simulink model "questao1"  (Simulink 3.00)
settings: Solver=ode45  StartTime=0.0  StopTime=4  RelTol=1e-3
settings Model: LastModifiedBy=Administrador

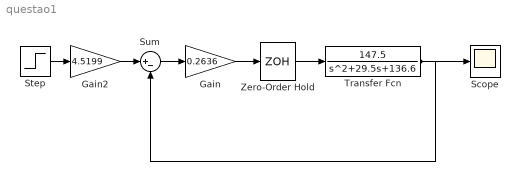
== system questao1 ==
  Gain : Gain  Gain=0.2636  SaturateOnIntegerOverflow=on
  Gain2 : Gain  Gain=4.5199  SaturateOnIntegerOverflow=on
  Scope : Scope
      settings: TimeRange=1.6  YMin=-5  YMax=5  SaveToWorkspace=off  SaveName=ScopeData
  Step : Step  Time=0  Before=0  After=1  SampleTime=0
  Sum : Sum  Inputs=|+-  SaturateOnIntegerOverflow=on
  Transfer Fcn : TransferFcn  Numerator=[147.5]  Denominator=[1 29.5 136.6]
  Zero-Order Hold : ZeroOrderHold  SampleTime=0.255
  wires:
  Sum/1 -> Gain/1
  Gain/1 -> Zero-Order Hold/1
  Zero-Order Hold/1 -> Transfer Fcn/1
  Transfer Fcn/1 -> Scope/1, Sum/2
  Step/1 -> Gain2/1
  Gain2/1 -> Sum/1
